simulink model "ChargeC22"  (R2020a)
settings: Solver=FixedStepAuto  StartTime=0.0  StopTime=10.0  FixedStep=1e-3  RelTol=1e-3  EnableMultiTasking=on
undefined symbols (not defined in the file): D5, PTA2
libraries: frdmk64flib x1
settings Model: ExtModeTrigDuration=5  Creator=WinnieTrandinh  LastModifiedBy=WinnieTrandinh
settings OptimizationCC: EnhancedBackFolding=on  PassReuseOutputArgsAs=Individual arguments  ZeroExternalMemoryAtStartup=off  ZeroInternalMemoryAtStartup=off  MaxStackSize=64  OptimizeBlockOrder=speed  DifferentSizesBufferReuse=on  OptimizationCustomize=off  EfficientTunableParamExpr=on
settings DebuggingCC: ParameterTunabilityLossMsg=error
settings HardwareCC: ProdBitPerPointer=32  ProdBitPerSizeT=32  ProdBitPerPtrDiffT=32  ProdLargestAtomicInteger=Long  ProdLargestAtomicFloat=Double  ProdWordSize=32  ProdHWDeviceType=ARM Compatible->ARM Cortex
settings SFSimCC: MATLABDynamicMemAlloc=off
settings RTWCC: SystemTargetFile=ert.tlc  HardwareBoard=NXP FRDM-K64F  TemplateMakefile=ert_default_tmf  Toolchain=GNU Tools for ARM Embedded Processors
settings CodeAppCC: ForceParamTrailComments=on  IgnoreCustomStorageClasses=off  OperatorAnnotations=on  SimulinkDataObjDesc=on  SFDataObjDesc=on  InsertBlockDesc=on

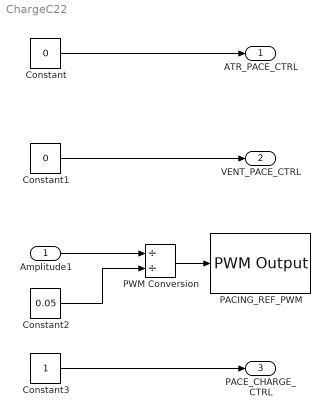
== system ChargeC22 ==
  Amplitude1 : Inport
  Constant : Constant  Value=0
  Constant1 : Constant  Value=0
  Constant2 : Constant  Value=0.05
  Constant3 : Constant
  PACING_REF_PWM : frdmk64flib/PWM Output  Priority=3  Whichpin=PTA2 (D5)  InitialFrequency=2000  InitialDutyCycle=20
  PWM Conversion : Product  Inputs=//
  ATR_PACE_CTRL : Outport
  VENT_PACE_CTRL : Outport  Port=2
  PACE_CHARGE_CTRL : Outport  Port=3
  wires:
  Constant/1 -> ATR_PACE_CTRL/1
  Constant1/1 -> VENT_PACE_CTRL/1
  Amplitude1/1 -> PWM Conversion/1
  PWM Conversion/1 -> PACING_REF_PWM/1
  Constant2/1 -> PWM Conversion/2
  Constant3/1 -> PACE_CHARGE_CTRL/1
